simulink model "diab_for_stat2__2016"  (R2016b)
settings: Solver=VariableStepAuto  StartTime=0.0  StopTime=25  RelTol=1e-6  EnableMultiTasking=on
undefined symbols (not defined in the file): normpdf
settings Model: Creator=Alex  LastModifiedBy=alex_
settings SolverCC: ZeroCrossAlgorithm=Adaptive
settings OptimizationCC: LifeSpan=inf
settings DebuggingCC: SFUnexpectedBacktrackingDiag=warning  SFNoUnconditionalDefaultTransitionDiag=warning  SFExecutionAtInitializationDiag=none
settings GRTTargetCC: TargetLangStandard=C89/C90 (ANSI)  GeneratePreprocessorConditionals=Disable all
settings ConfigComp: CovMetricSettings=dw  CovHtmlReporting=on  CovSaveCumulativeToWorkspaceVar=on  CovSaveSingleToWorkspaceVar=on  CovExternalEMLEnable=off

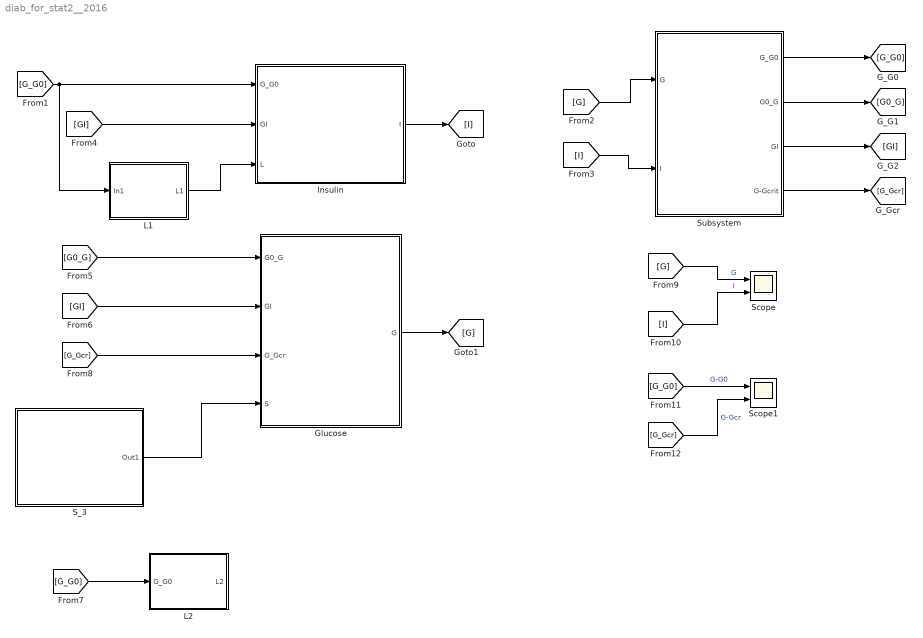
== system diab_for_stat2__2016 ==
  Glucose : Subsystem
  Insulin : Subsystem
  L1 : Subsystem
  L2 : Subsystem
  S_3 : Subsystem
  Scope : Scope  NumInputPorts=2
  Scope1 : Scope  NumInputPorts=2
  Subsystem : Subsystem
  wires:
  [I] -> Scope/2  "I"
  [G] -> Scope/1  "G"
  [G_G0] -> Scope1/1  "G-G0"
  [G_Gcr] -> Scope1/2  "G-Gcr"
  [G] -> Subsystem/1(G)
  [I] -> Subsystem/2(I)
  Subsystem/1(G_G0) -> [G_G0]
  Subsystem/2(G0_G) -> [G0_G]
  Subsystem/3(GI) -> [GI]
  Subsystem/4(G-Gcrit) -> [G_Gcr]
  [G_G0] -> L1/1(In1), Insulin/1(G_G0)
  [GI] -> Insulin/2(GI)
  L1/1(L1) -> Insulin/3(L)
  Insulin/1(I) -> [I]
  [G0_G] -> Glucose/1(G0_G)
  [GI] -> Glucose/2(GI)
  [G_Gcr] -> Glucose/3(G_Gcr)
  S_3/1(Out1) -> Glucose/4(S)
  Glucose/1(G) -> [G]
  [G_G0] -> L2/1(G_G0)

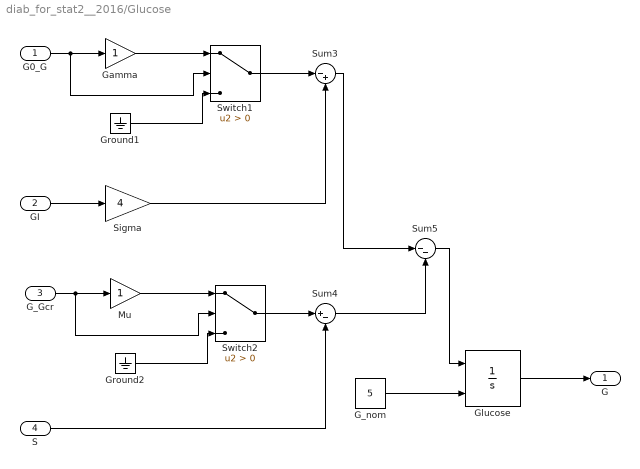
== system diab_for_stat2__2016/Glucose ==
  G0_G : Inport
  GI : Inport  Port=2
  G_Gcr : Inport  Port=3
  S : Inport  Port=4
  G_nom : Constant  Value=5
  Gamma : Gain
  Glucose : Integrator  InitialConditionSource=external
  Ground1 : Ground
  Ground2 : Ground
  Mu : Gain
  Sigma : Gain  Gain=4
  Sum3 : Sum  Inputs=|-+
  Sum4 : Sum  Inputs=|+-
  Sum5 : Sum  Inputs=|--
  Switch1 : Switch  Criteria=u2 > Threshold
  Switch2 : Switch  Criteria=u2 > Threshold
  G : Outport
  wires:
  Ground1/1 -> Switch1/3
  Gamma/1 -> Switch1/1
  Sum4/1 -> Sum5/2
  Sigma/1 -> Sum3/2
  S/1 -> Sum4/2
  G_Gcr/1 -> Switch2/2, Mu/1
  G_nom/1 -> Glucose/2
  Mu/1 -> Switch2/1
  Switch2/1 -> Sum4/1
  Ground2/1 -> Switch2/3
  Switch1/1 -> Sum3/1
  Sum3/1 -> Sum5/1
  G0_G/1 -> Gamma/1, Switch1/2
  Sum5/1 -> Glucose/1
  Glucose/1 -> G/1
  GI/1 -> Sigma/1

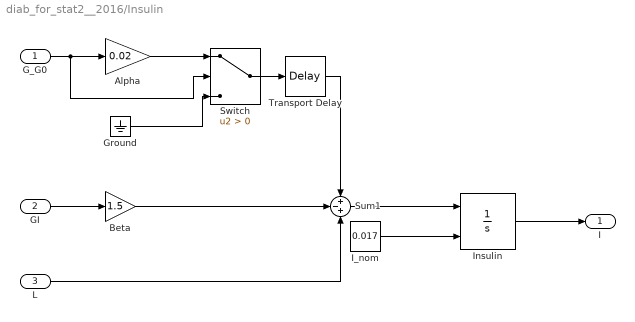
== system diab_for_stat2__2016/Insulin ==
  G_G0 : Inport
  GI : Inport  Port=2
  L : Inport  Port=3
  Alpha : Gain  Gain=0.02
  Beta : Gain  Gain=1.5
  Ground : Ground
  I_nom : Constant  Value=0.017
  Insulin : Integrator  InitialConditionSource=external
  Sum1 : Sum  Inputs=+-+
  Switch : Switch  Criteria=u2 > Threshold
  Transport Delay : TransportDelay  DelayTime=0.5
  I : Outport
  wires:
  I_nom/1 -> Insulin/2
  Beta/1 -> Sum1/2
  Alpha/1 -> Switch/1
  Sum1/1 -> Insulin/1
  Ground/1 -> Switch/3
  G_G0/1 -> Switch/2, Alpha/1
  GI/1 -> Beta/1
  Switch/1 -> Transport Delay/1
  Insulin/1 -> I/1
  L/1 -> Sum1/3
  Transport Delay/1 -> Sum1/1

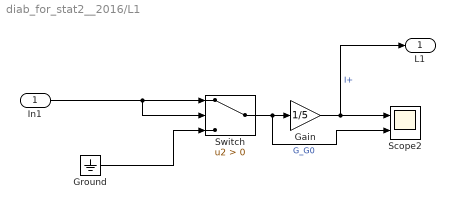
== system diab_for_stat2__2016/L1 ==
  In1 : Inport
  Gain : Gain  Gain=1/5
  Ground : Ground
  Scope2 : Scope  NumInputPorts=2
  Switch : Switch  Criteria=u2 > Threshold
  L1 : Outport
  wires:
  Switch/1 -> Scope2/2, Gain/1  "G_G0"
  In1/1 -> Switch/2, Switch/1
  Gain/1 -> L1/1, Scope2/1  "I+"
  Ground/1 -> Switch/3

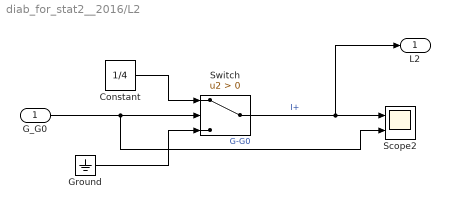
== system diab_for_stat2__2016/L2 ==
  G_G0 : Inport
  Constant : Constant  Value=1/4
  Ground : Ground
  Scope2 : Scope  NumInputPorts=2
  Switch : Switch  Criteria=u2 > Threshold
  L2 : Outport
  wires:
  Ground/1 -> Switch/3
  G_G0/1 -> Scope2/2, Switch/2  "G-G0"
  Switch/1 -> Scope2/1, L2/1  "I+"
  Constant/1 -> Switch/1

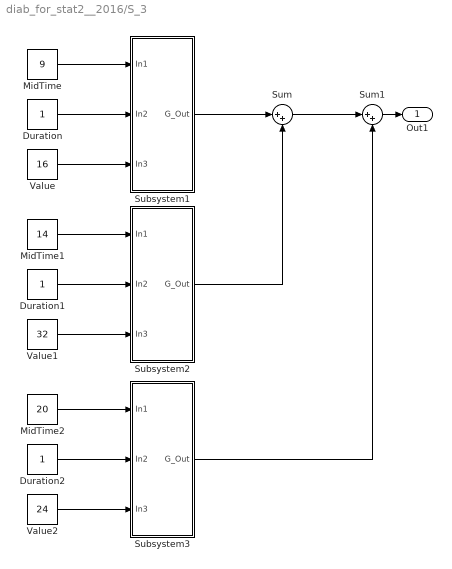
== system diab_for_stat2__2016/S_3 ==
  Duration : Constant
  Duration1 : Constant
  Duration2 : Constant
  MidTime : Constant  Value=9
  MidTime1 : Constant  Value=14
  MidTime2 : Constant  Value=20
  Subsystem1 : Subsystem
  Subsystem2 : Subsystem
  Subsystem3 : Subsystem
  Sum : Sum  Inputs=|++
  Sum1 : Sum  Inputs=|++
  Value : Constant  Value=16
  Value1 : Constant  Value=32
  Value2 : Constant  Value=24
  Out1 : Outport
  wires:
  Value2/1 -> Subsystem3/3(In3)
  Duration2/1 -> Subsystem3/2(In2)
  MidTime2/1 -> Subsystem3/1(In1)
  Duration/1 -> Subsystem1/2(In2)
  Value/1 -> Subsystem1/3(In3)
  Subsystem1/1(G_Out) -> Sum/1
  Subsystem2/1(G_Out) -> Sum/2
  MidTime/1 -> Subsystem1/1(In1)
  Sum/1 -> Sum1/1
  Subsystem3/1(G_Out) -> Sum1/2
  Value1/1 -> Subsystem2/3(In3)
  MidTime1/1 -> Subsystem2/1(In1)
  Duration1/1 -> Subsystem2/2(In2)
  Sum1/1 -> Out1/1

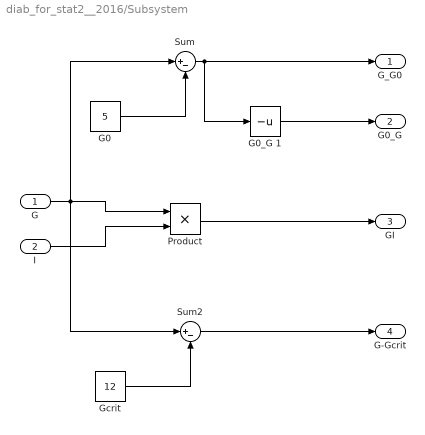
== system diab_for_stat2__2016/Subsystem ==
  G : Inport
  I : Inport  Port=2
  G0 : Constant  Value=5
  G0_G 1 : UnaryMinus
  Gcrit : Constant  Value=12
  Product : Product
  Sum : Sum  Inputs=|+-
  Sum2 : Sum  Inputs=|+-
  G_G0 : Outport
  G0_G : Outport  Port=2
  GI : Outport  Port=3
  G-Gcrit : Outport  Port=4
  wires:
  G0/1 -> Sum/2
  Sum/1 -> G_G0/1, G0_G 1/1
  Gcrit/1 -> Sum2/2
  I/1 -> Product/2
  Sum2/1 -> G-Gcrit/1
  G/1 -> Sum2/1, Sum/1, Product/1
  G0_G 1/1 -> G0_G/1
  Product/1 -> GI/1

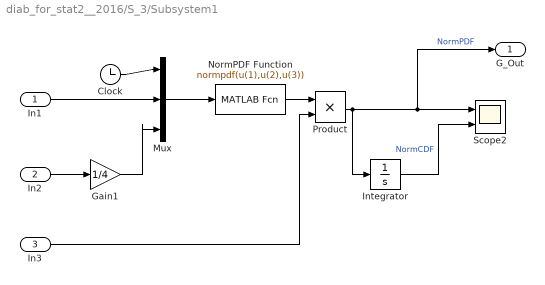
== system diab_for_stat2__2016/S_3/Subsystem1 ==
  In1 : Inport
  In2 : Inport  Port=2
  In3 : Inport  Port=3
  Clock : Clock
  Gain1 : Gain  Gain=1/4
  Integrator : Integrator
  Mux : Mux  Inputs=3
  NormPDF Function : MATLABFcn  MATLABFcn=normpdf(u(1),u(2),u(3))
  Product : Product
  Scope2 : Scope  NumInputPorts=2
  G_Out : Outport
  wires:
  In2/1 -> Gain1/1
  Product/1 -> Integrator/1, G_Out/1, Scope2/1  "NormPDF"
  Gain1/1 -> Mux/3
  Clock/1 -> Mux/1
  In1/1 -> Mux/2
  NormPDF Function/1 -> Product/1
  Integrator/1 -> Scope2/2  "NormCDF"
  Mux/1 -> NormPDF Function/1
  In3/1 -> Product/2

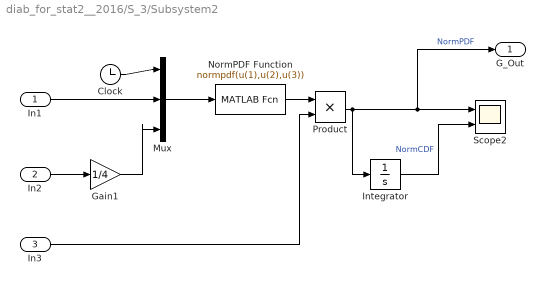
== system diab_for_stat2__2016/S_3/Subsystem2 ==
  In1 : Inport
  In2 : Inport  Port=2
  In3 : Inport  Port=3
  Clock : Clock
  Gain1 : Gain  Gain=1/4
  Integrator : Integrator
  Mux : Mux  Inputs=3
  NormPDF Function : MATLABFcn  MATLABFcn=normpdf(u(1),u(2),u(3))
  Product : Product
  Scope2 : Scope  NumInputPorts=2
  G_Out : Outport
  wires:
  In3/1 -> Product/2
  Mux/1 -> NormPDF Function/1
  Integrator/1 -> Scope2/2  "NormCDF"
  NormPDF Function/1 -> Product/1
  In1/1 -> Mux/2
  Clock/1 -> Mux/1
  Gain1/1 -> Mux/3
  Product/1 -> Scope2/1, G_Out/1, Integrator/1  "NormPDF"
  In2/1 -> Gain1/1

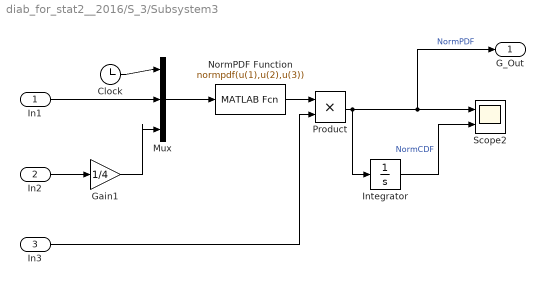
== system diab_for_stat2__2016/S_3/Subsystem3 ==
  In1 : Inport
  In2 : Inport  Port=2
  In3 : Inport  Port=3
  Clock : Clock
  Gain1 : Gain  Gain=1/4
  Integrator : Integrator
  Mux : Mux  Inputs=3
  NormPDF Function : MATLABFcn  MATLABFcn=normpdf(u(1),u(2),u(3))
  Product : Product
  Scope2 : Scope  NumInputPorts=2
  G_Out : Outport
  wires:
  In2/1 -> Gain1/1
  Product/1 -> Integrator/1, G_Out/1, Scope2/1  "NormPDF"
  Gain1/1 -> Mux/3
  Clock/1 -> Mux/1
  In1/1 -> Mux/2
  NormPDF Function/1 -> Product/1
  Integrator/1 -> Scope2/2  "NormCDF"
  Mux/1 -> NormPDF Function/1
  In3/1 -> Product/2
